simulink model "model_based_project_plant_simulink"  (R2024b)
settings: Solver=VariableStepAuto  StartTime=0.0  StopTime=5  RelTol=1e-3
settings Model: Creator=sueda  LastModifiedBy=sueda

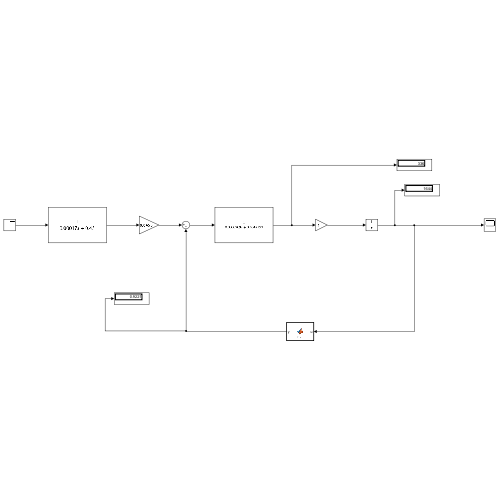
[thumbnail: Simulink's stored preview of the top-level diagram]
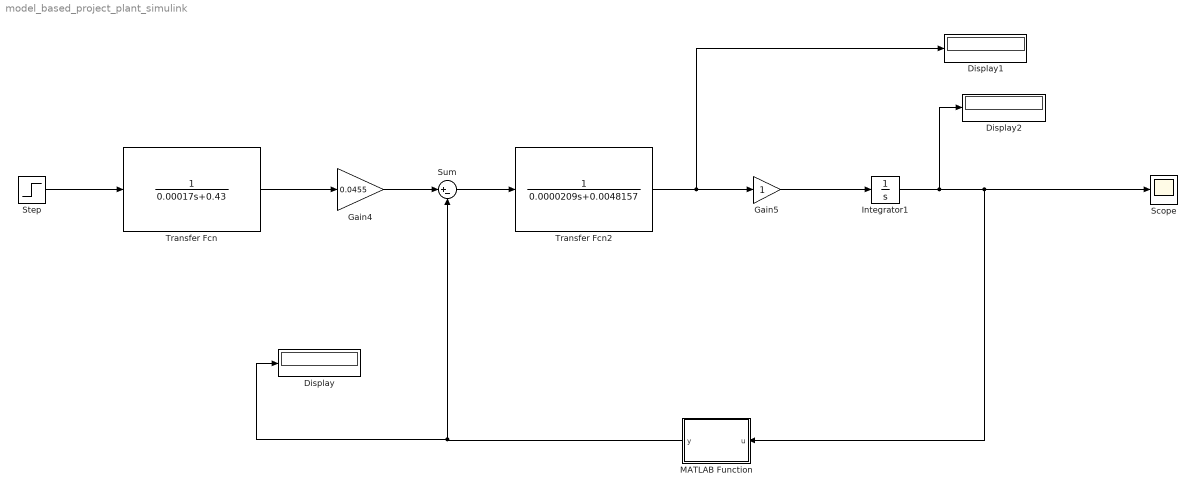
== system model_based_project_plant_simulink ==
  Display : Display
  Display1 : Display
  Display2 : Display
  Gain4 : Gain  Gain=0.0455
  Gain5 : Gain
  Integrator1 : Integrator
  MATLAB Function : MATLAB Function  TreatAsAtomicUnit=on
  Scope : Scope
  Step : Step  After=24  SampleTime=0
  Sum : Sum  Inputs=|+-
  Transfer Fcn : TransferFcn  Denominator=[0.00017 0.43]
  Transfer Fcn2 : TransferFcn  Denominator=[0.0000209 0.0048157]
  wires:
  Step/1 -> Transfer Fcn/1
  Transfer Fcn2/1 -> Display1/1, Gain5/1
  Gain5/1 -> Integrator1/1
  Transfer Fcn/1 -> Gain4/1
  Gain4/1 -> Sum/1
  Sum/1 -> Transfer Fcn2/1
  Integrator1/1 -> Display2/1, MATLAB Function/1(u), Scope/1
  MATLAB Function/1(y) -> Display/1, Sum/2

== matlab function model_based_project_plant_simulink/MATLAB Function ==
  data: u input; y output
function y = fcn(u)

y = 0.0005*u+0.1;
